simulink model "cartpole_lqr_simulink"  (R2025a)
settings: Solver=ode45  StartTime=0.0  StopTime=10  MaxStep=0.001  RelTol=1e-3
values from neighbouring files (symbols this model uses):
  Fmax = 50    [auto_tune_pid.m]    (also in setup_lqr.m; setup_pd.m; setup_pid.m)
  K = lqr(A, B, Q, R)    [setup_lqr.m]
settings Model: Creator=Lee  LastModifiedBy=Lee

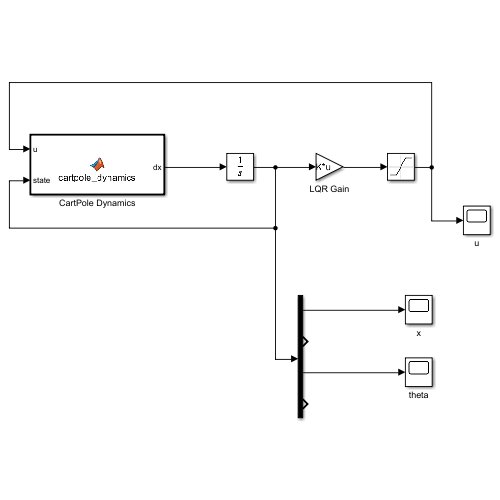
[thumbnail: Simulink's stored preview of the top-level diagram]
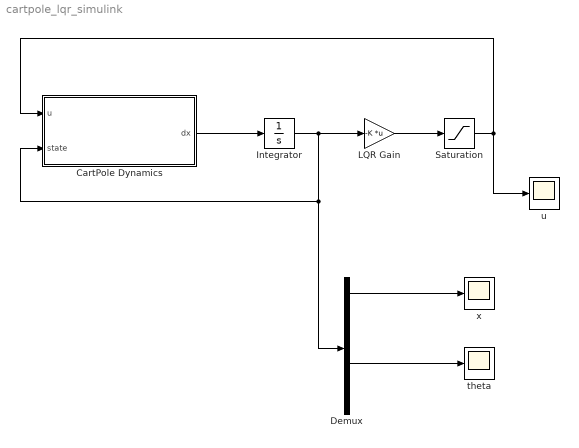
== system cartpole_lqr_simulink ==
  CartPole Dynamics : MATLAB Function  TreatAsAtomicUnit=on
  Demux : Demux
  Integrator : Integrator  InitialCondition=[0; 0; deg2rad(5); 0]
  LQR Gain : Gain  Gain=-K  Multiplication=Matrix(K*u)
  Saturation : Saturate  UpperLimit=Fmax  LowerLimit=-Fmax
  theta : Scope
      settings: ActiveDisplayYMinimum=-0.038361494220970779  ActiveDisplayYMaximum=0.10122512446868173
  u : Scope
      settings: ActiveDisplayYMinimum=-1.6622560436908524  ActiveDisplayYMaximum=9.0323745598358371  DataLoggingVariableName=ScopeData2
  x : Scope
      settings: ActiveDisplayYMinimum=-0.017316307064661942  ActiveDisplayYMaximum=0.12743512539960761
  wires:
  CartPole Dynamics/1(dx) -> Integrator/1
  Integrator/1 -> CartPole Dynamics/2(state), Demux/1, LQR Gain/1
  LQR Gain/1 -> Saturation/1
  Saturation/1 -> u/1, CartPole Dynamics/1(u)
  Demux/1 -> x/1
  Demux/3 -> theta/1

== matlab function cartpole_lqr_simulink/CartPole Dynamics ==
  data: u input; dx output; state input
function dx = cartpole_dynamics(u, state)

M = 1.0;
m = 0.1;
l = 0.5;
g = 9.8;

x = state(1);
x_dot = state(2);
theta = state(3);
theta_dot = state(4);

den = M + m*sin(theta)^2;

x_ddot = (u + m * sin(theta) * (l * theta_dot^2 - g * cos(theta))) / den;

theta_ddot = (-u * cos(theta) - m * l * theta_dot^2 * sin(theta) * cos(theta) + (M + m) * g * sin(theta)) / (l * den);

dx = zeros(4,1);
dx(1) = x_dot;
dx(2) = x_ddot;
dx(3) = theta_dot;
dx(4) = theta_ddot;

end
